simulink model "L02_TrafficLight"  (R2020b)
settings: Solver=FixedStepAuto  StartTime=0.0  StopTime=300  FixedStep=1  RelTol=1e-3
undefined symbols (not defined in the file): sigbuilder_block
settings Model: Creator=Nic  LastModifiedBy=Nic

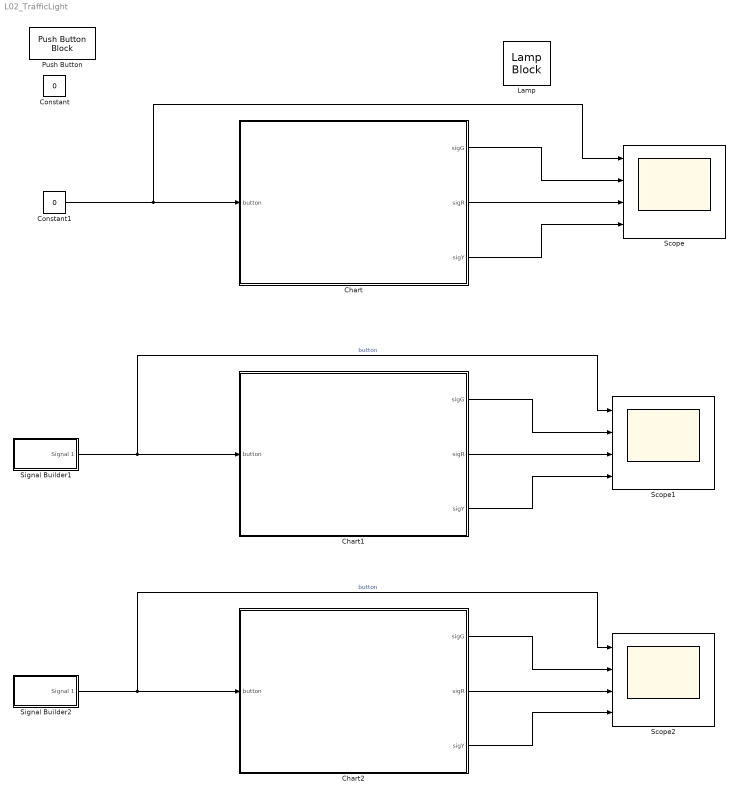
== system L02_TrafficLight ==
  Chart : Stateflow chart  TreatAsAtomicUnit=on
  Chart1 : Stateflow chart  TreatAsAtomicUnit=on
  Chart2 : Stateflow chart  TreatAsAtomicUnit=on
  Constant : Constant  Value=0
  Constant1 : Constant  Value=0
  Lamp : LampBlock
  Push Button : PushButtonBlock
  Scope : Scope  NumInputPorts=4
  Scope1 : Scope  NumInputPorts=4
  Scope2 : Scope  NumInputPorts=4
  Signal Builder1 : Subsystem  Tag=STV Subsys  LoadFcn=sigbuilder_block('load');  StartFcn=sigbuilder_block('start');  StopFcn=sigbuilder_block('stop');  ClipboardFcn=sigbuilder_block('clipboard');  mask(Sigbuilder block){tuvar=[0:10]}
      mask help: Simulink:masks:SigbuilderBlock_MD
      mask init:
      | if ~strcmp(get_param(bdroot(gcbh),'SimulationStatus'),'stopped') tuvar = sigbuilder_block('maskInit'); end
      settings: CopyFcn=sigbuilder_block('copy');  DeleteFcn=sigbuilder_block('delete');  ModelCloseFcn=sigbuilder_block('modelClose');  PreSaveFcn=sigbuilder_block('preSave');  PauseFcn=sigbuilder_block('pause');  ContinueFcn=sigbuilder_block('continue');  NameChangeFcn=sigbuilder_block('namechange');  OpenFcn=sigbuilder_block('open',[142.8 98.4 888 400.2 ]);  CloseFcn=sigbuilder_block('close');
      mask Display: plot(0, 0, 100, 100,[2, 2, 32, 32, 2], [68, 8, 8, 68, 68],[32, 2], [38, 38], [32, 19, 2],[53, 60, 44], [32, 17, 17, 2],[16, 16, 31, 31]);txt = getActiveGroup(gcbh);text(2, 100, txt,'verticalAlignment', 'top');
  Signal Builder2 : Subsystem  Tag=STV Subsys  LoadFcn=sigbuilder_block('load');  StartFcn=sigbuilder_block('start');  StopFcn=sigbuilder_block('stop');  ClipboardFcn=sigbuilder_block('clipboard');  mask(Sigbuilder block){tuvar=[0:10]}
      mask help: Simulink:masks:SigbuilderBlock_MD
      mask init:
      | if ~strcmp(get_param(bdroot(gcbh),'SimulationStatus'),'stopped') tuvar = sigbuilder_block('maskInit'); end
      settings: CopyFcn=sigbuilder_block('copy');  DeleteFcn=sigbuilder_block('delete');  ModelCloseFcn=sigbuilder_block('modelClose');  PreSaveFcn=sigbuilder_block('preSave');  PauseFcn=sigbuilder_block('pause');  ContinueFcn=sigbuilder_block('continue');  NameChangeFcn=sigbuilder_block('namechange');  OpenFcn=sigbuilder_block('open',[142.8 98.4 888 400.2 ]);  CloseFcn=sigbuilder_block('close');
      mask Display: plot(0, 0, 100, 100,[2, 2, 32, 32, 2], [68, 8, 8, 68, 68],[32, 2], [38, 38], [32, 19, 2],[53, 60, 44], [32, 17, 17, 2],[16, 16, 31, 31]);txt = getActiveGroup(gcbh);text(2, 100, txt,'verticalAlignment', 'top');
  wires:
  Chart/1(sigG) -> Scope/2
  Chart/2(sigR) -> Scope/3
  Chart/3(sigY) -> Scope/4
  Constant1/1 -> Scope/1, Chart/1(button)
  Chart1/3(sigY) -> Scope1/4
  Chart1/2(sigR) -> Scope1/3
  Chart1/1(sigG) -> Scope1/2
  Signal Builder1/1(Signal 1) -> Scope1/1, Chart1/1(button)  "button"
  Signal Builder2/1(Signal 1) -> Chart2/1(button), Scope2/1  "button"
  Chart2/1(sigG) -> Scope2/2
  Chart2/2(sigR) -> Scope2/3
  Chart2/3(sigY) -> Scope2/4

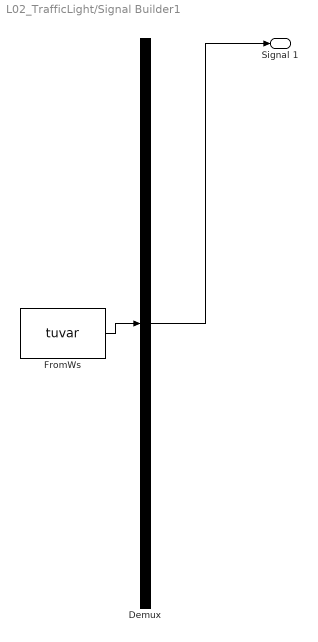
== system L02_TrafficLight/Signal Builder1 ==
  Demux : Demux  Tag=STV Demux  Outputs=1
      settings: DisplayOption=none
  FromWs : FromWorkspace  Tag=STV FromWs  VariableName=tuvar
      SigBuilderData=|
      | common.afterFinalStr = 'Extrapolate'
      | common.sampleTime = 0
      | dataSet.timeRange = [0 100]
      | dataSet.name = 'Group 1'
      | sbobj.Groups.Name = 'Group 1'
      | sbobj.Groups.Signals.Name = 'Signal 1'
      | sbobj.Groups.Signals.XData = [0 47.9 47.9 50 50 100]
      | sbobj.Groups.Signals.YData = [0 0 1 1 0 0]
      | sbobj.Groups.TimeRange = [0 100]
  Signal 1 : Outport  Tag=STV Outport
  wires:
  FromWs/1 -> Demux/1
  Demux/1 -> Signal 1/1

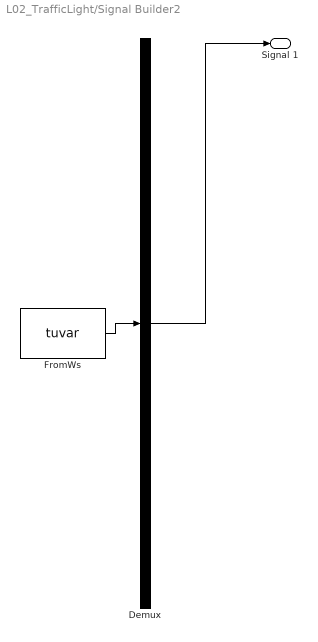
== system L02_TrafficLight/Signal Builder2 ==
  Demux : Demux  Tag=STV Demux  Outputs=1
      settings: DisplayOption=none
  FromWs : FromWorkspace  Tag=STV FromWs  VariableName=tuvar
      SigBuilderData=|
      | common.afterFinalStr = 'Extrapolate'
      | common.sampleTime = 0
      | dataSet.timeRange = [0 150]
      | dataSet.name = 'Group 1'
      | sbobj.Groups.Name = 'Group 1'
      | sbobj.Groups.Signals.Name = 'Signal 1'
      | sbobj.Groups.Signals.XData = [0 113.4 113.4 140.6 140.6 150]
      | sbobj.Groups.Signals.YData = [0 0 1 1 0 0]
      | sbobj.Groups.TimeRange = [0 150]
  Signal 1 : Outport  Tag=STV Outport
  wires:
  Demux/1 -> Signal 1/1
  FromWs/1 -> Demux/1

== stateflow chart L02_TrafficLight/Chart1 ==
  state RED
    en:
    sigR = true;
    sigY = false;
    sigG = false;
  state YELLOW
    en:
    sigR = false;
    sigY = true;
    sigG = false;
  state GREEN_NOT_PRESSED
    en:
    sigR = false;
    sigY = false;
    sigG = true;
  state GREEN_PRESSED
  state GREEN [commented out]
    entry:
    sigR = false;
    sigY = false;
    sigG = true;
    state GREEN_NOT_PRESSED [commented out]
    state GREEN_PRESSED [commented out]
    (default) -> GREEN.GREEN_NOT_PRESSED [commented out]
    GREEN.GREEN_NOT_PRESSED -> GREEN.GREEN_PRESSED [commented out] : [button == true]
        | {ButtonPressed = true;}
  (default) -> RED
  YELLOW -> RED : [after(5, sec)]
  GREEN_NOT_PRESSED -> YELLOW [order 1] : [count >= 60 && button == true]
  GREEN_PRESSED -> YELLOW [order 1] : [count >= 60]
  RED -> GREEN_NOT_PRESSED : [after(30, sec)]
      | {%ButtonPressed=false;
      | count = 0;}
  GREEN_NOT_PRESSED -> GREEN_PRESSED [order 2] : [button == true]
      | {count = count+1;}
  GREEN_NOT_PRESSED -> GREEN_NOT_PRESSED [order 3] : {count=count+1;}
  GREEN_PRESSED -> GREEN_PRESSED [order 2] : {count = count+1;}
  data: button input; sigG output; sigR output; sigY output; count local

== stateflow chart L02_TrafficLight/Chart2 ==
  state RED
    en:
    sigR = true;
    sigY = false;
    sigG = false;
  state YELLOW
    en:
    sigR = false;
    sigY = true;
    sigG = false;
  state GREEN_NOT_PRESSED
    en:
    sigR = false;
    sigY = false;
    sigG = true;
  state GREEN_PRESSED
  state GREEN [commented out]
    entry:
    sigR = false;
    sigY = false;
    sigG = true;
    state GREEN_NOT_PRESSED [commented out]
    state GREEN_PRESSED [commented out]
    (default) -> GREEN.GREEN_NOT_PRESSED [commented out]
    GREEN.GREEN_NOT_PRESSED -> GREEN.GREEN_PRESSED [commented out] : [button == true]
        | {ButtonPressed = true;}
  (default) -> RED
  YELLOW -> RED : [after(5, sec)]
  GREEN_NOT_PRESSED -> YELLOW [order 1] : [count >= 60 && button == true]
  GREEN_PRESSED -> YELLOW [order 1] : [count >= 60]
  RED -> GREEN_NOT_PRESSED : [after(30, sec)]
      | {%ButtonPressed=false;
      | count = 0;}
  GREEN_NOT_PRESSED -> GREEN_PRESSED [order 2] : [button == true]
      | {count = count+1;}
  GREEN_NOT_PRESSED -> GREEN_NOT_PRESSED [order 3] : {count=count+1;}
  GREEN_PRESSED -> GREEN_PRESSED [order 2] : {count = count+1;}
  data: button input; sigG output; sigR output; sigY output; count local

== stateflow chart L02_TrafficLight/Chart ==
  state RED
    en:
    sigR = true;
    sigY = false;
    sigG = false;
  state YELLOW
    en:
    sigR = false;
    sigY = true;
    sigG = false;
  state GREEN_NOT_PRESSED
    en:
    sigR = false;
    sigY = false;
    sigG = true;
  state GREEN_PRESSED
  state GREEN [commented out]
    entry:
    sigR = false;
    sigY = false;
    sigG = true;
    state GREEN_NOT_PRESSED [commented out]
    state GREEN_PRESSED [commented out]
    (default) -> GREEN.GREEN_NOT_PRESSED [commented out]
    GREEN.GREEN_NOT_PRESSED -> GREEN.GREEN_PRESSED [commented out] : [button == true]
        | {ButtonPressed = true;}
  (default) -> RED
  YELLOW -> RED : [after(5, sec)]
  GREEN_NOT_PRESSED -> YELLOW [order 1] : [count >= 60 && button == true]
  GREEN_PRESSED -> YELLOW [order 1] : [count >= 60]
  RED -> GREEN_NOT_PRESSED : [after(30, sec)]
      | {%ButtonPressed=false;
      | count = 0;}
  GREEN_NOT_PRESSED -> GREEN_PRESSED [order 2] : [button == true]
      | {count = count+1;}
  GREEN_NOT_PRESSED -> GREEN_NOT_PRESSED [order 3] : {count=count+1;}
  GREEN_PRESSED -> GREEN_PRESSED [order 2] : {count = count+1;}
  data: button input; sigG output; sigR output; sigY output; count local
